simulink model "NonlinearMPC_FL_CBFcontroller"  (R2026a)
settings: Solver=VariableStepAuto  StopTime=120
PreLoadFcn:
  | % Define variants
  | VSS_PATH_CTRL_PURE_PURSUIT=Simulink.Variant('VSS_PATH_CTRL_MODE==1');
  | VSS_PATH_CTRL_REAR_WHEEL=Simulink.Variant('VSS_PATH_CTRL_MODE==2');
  | % Select default variant
  | VSS_PATH_CTRL_MODE =1;
  | 
  | 
  | % Longitudinal PID
  | LongitudinalPID.Kp = 20;
  | LongitudinalPID.Ki = 0;
  | LongitudinalPID.Kd = 0;
  | LongitudinalPID.N = 100;
  | LongitudinalPID.MaxAccel = 80;
  | LongitudinalPID.SampleTime = 0.01;
  | 
  | % Steering PID
  | SteeringPID.Kp = 60;
  | SteeringPID.Ki = 0;
  | SteeringPID.Kd = 5;
  | SteeringPID.N = 10;
  | SteeringPID.MaxSpeed =  10;
  | SteeringPID.MinSpeed = -10;
  | SteeringPID.SampleTime = 0.01;
  | 
  | 
  | 
  | setSMVehicleVisuParameters;
  | 
  | % Load planner commands
  | load('PlannerCmdTests.mat');
  | % Assign one for testing:
  | plannerCmd = plannerCmdFwd;
  | % plannerCmd  = plannerCmdFwdBwd;
  | 
  | % Bus structure definition
  | load('PlannerBusStruct.mat');
  | 
  | % Rear Wheel Controller Parameters
  | RW.k_e = 0.2;    % 0.1
  | RW.k_theta = 1;   % 0.75
  | RW.SampleTime =  0.1;
  | RW.GoalRadius = 0.3;
  | 
  | % Pure pursuit parameters
  | PP.DesiredLinearVel = 5;
  | PP.MaxAngularVel  = 10;
  | PP.LookaheadDist  = 1;
  | PP.Wheelbase = 4;
  | PP.GoalRadius = 0.1;
  | PP.SampleTime = 0.1;
  | PP.LongitudinalPID.Kp = 20;
  | PP.LongitudinalPID.Ki = 0;
  | PP.LongitudinalPID.Kd = 0;
  | PP.LongitudinalPID.N = 100;
  | PP.LongitudinalPID.MaxLongAccel =  80;
  | PP.LongitudinalPID.MinLongAccel = -80;
  | 
  | % Spline ref
  | splineRef = [ 0 0 0;[plannerCmd.PathMatrix(1:plannerCmd.PathLengths(1),1:2,1),0*ones(length(plannerCmd.PathMatrix(1:plannerCmd.PathLengths(1),1,1)),1)]];
values from neighbouring files (symbols this model uses):
  m = max(2, ceil(Lseg/ds))    [Trajectory.m]    (also in plot_nmpc_result.m = NaN)
  s = [0; cumsum(hypot(diff(xs),diff(ys)))]    [Trajectory.m]    (also in plot_parking_mpc.m = evalin('base',name); plot_result.m = out.(names{k}))
  trajMatrix = [tvec, xd, yd, thd, vd, wd]    [Trajectory.m]    (also in plot_parking_mpc.m = evalin('base','trajMatrix'); plot_result.m = evalin('base','trajMatrix'))
undefined symbols (not defined in the file or in its folder): DiscIntNeverNeededParam, smvv, X, Y, Z
libraries: sm_lib x527, sm_vehicle_slalom_lib x48, fl_lib x40, fl_ps_legacy_lib x28, nesl_utility x13
(part 15 of 15)

== system NonlinearMPC_FL_CBFcontroller/Robot Bicycle Model/Visualizer/SM_Car_Visu/Vehicle7/Steering_Wheel/Logo/LStick3 ==
  Stick : sm_lib/Body Elements/Brick Solid  BrickDimensions=[smvv.steeringwheel.letterStick 0.001 0.001]  BrickDimensionsUnits=m  ExportEntireGeometry=off  InertiaType=PointMass  BasedOnType=Density  Density=1000  DensityUnits=kg/m^3  Mass=0.001  MassUnits=kg  CenterOfMass=[0 0 0]  CenterOfMassUnits=m  MomentsOfInertia=[1 1 1]  MomentsOfInertiaUnits=kg*m^2  ProductsOfInertia=[1 1 1]  ProductsOfInertiaUnits=kg*m^2  GraphicType=FromGeometry  MarkerShape=Sphere  MarkerSize=10  GraphicVisPropType=SimpleVisualProperties  GraphicDiffuseColor=smvv.steeringwheel.letterColor  GraphicOpacity=1.0  GraphicSpecularColor=[0.5 0.5 0.5 1.0]  GraphicAmbientColor=[0.15 0.15 0.15 1.0]  GraphicEmissiveColor=[0.0 0.0 0.0 1.0]  GraphicShininess=75  DoExposeReferenceFrame=on  SerializedFrames=<Frames/>
  X offset 1 : sm_lib/Frames and Transforms/Rigid Transform  RotationMethod=None  FollAlignAxisA=+X  BaseAlignAxisA=+Y  FollAlignAxisB=+Y  BaseAlignAxisB=+Z  RotationStandardAxis=+X  RotationAngle=0  RotationAngleUnits=deg  RotationArbitraryAxis=[0 0 1]  RotationSequenceAxes=FollowerAxes  RotationSequence=XYX  RotationSequenceAngles=[0 0 0]  RotationSequenceAnglesUnits=deg  RotationMatrix=[1 0 0; 0 1 0; 0 0 1]  Quaternion=[1 0 0 0]  TranslationMethod=StandardAxis  TranslationCartesianOffset=[0 0 0]  TranslationCartesianOffsetUnits=m  TranslationStandardAxis=-X  TranslationStandardOffset=0.5*smvv.steeringwheel.letterStick  TranslationStandardOffsetUnits=m  TranslationROffset=0  TranslationROffsetUnits=m  TranslationThetaOffset=0  TranslationThetaOffsetUnits=deg  TranslationZOffset=0  TranslationZOffsetUnits=m
  x offset 2 : sm_lib/Frames and Transforms/Rigid Transform  RotationMethod=None  FollAlignAxisA=+X  BaseAlignAxisA=+Y  FollAlignAxisB=+Y  BaseAlignAxisB=+Z  RotationStandardAxis=+X  RotationAngle=0  RotationAngleUnits=deg  RotationArbitraryAxis=[0 0 1]  RotationSequenceAxes=FollowerAxes  RotationSequence=XYX  RotationSequenceAngles=[0 0 0]  RotationSequenceAnglesUnits=deg  RotationMatrix=[1 0 0; 0 1 0; 0 0 1]  Quaternion=[1 0 0 0]  TranslationMethod=StandardAxis  TranslationCartesianOffset=[0 0 0]  TranslationCartesianOffsetUnits=m  TranslationStandardAxis=+X  TranslationStandardOffset=0.5*smvv.steeringwheel.letterStick  TranslationStandardOffsetUnits=m  TranslationROffset=0  TranslationROffsetUnits=m  TranslationThetaOffset=0  TranslationThetaOffsetUnits=deg  TranslationZOffset=0  TranslationZOffsetUnits=m
  Conn1 : PMIOPort  Side=Left
  Conn2 : PMIOPort  Port=2  Side=Right
  connections:
  X offset 1/RConn1 -- Conn1/RConn1
  x offset 2/RConn1 -- Conn2/RConn1
  x offset 2/LConn1 -- Stick/RConn1 -- X offset 1/LConn1

== system NonlinearMPC_FL_CBFcontroller/Robot Bicycle Model/Visualizer/SM_Car_Visu/Vehicle7/Steering_Wheel/Logo/LStick4 ==
  Stick : sm_lib/Body Elements/Brick Solid  BrickDimensions=[smvv.steeringwheel.letterStick 0.001 0.001]  BrickDimensionsUnits=m  ExportEntireGeometry=off  InertiaType=PointMass  BasedOnType=Density  Density=1000  DensityUnits=kg/m^3  Mass=0.001  MassUnits=kg  CenterOfMass=[0 0 0]  CenterOfMassUnits=m  MomentsOfInertia=[1 1 1]  MomentsOfInertiaUnits=kg*m^2  ProductsOfInertia=[1 1 1]  ProductsOfInertiaUnits=kg*m^2  GraphicType=FromGeometry  MarkerShape=Sphere  MarkerSize=10  GraphicVisPropType=SimpleVisualProperties  GraphicDiffuseColor=smvv.steeringwheel.letterColor  GraphicOpacity=1.0  GraphicSpecularColor=[0.5 0.5 0.5 1.0]  GraphicAmbientColor=[0.15 0.15 0.15 1.0]  GraphicEmissiveColor=[0.0 0.0 0.0 1.0]  GraphicShininess=75  DoExposeReferenceFrame=on  SerializedFrames=<Frames/>
  X offset 1 : sm_lib/Frames and Transforms/Rigid Transform  RotationMethod=None  FollAlignAxisA=+X  BaseAlignAxisA=+Y  FollAlignAxisB=+Y  BaseAlignAxisB=+Z  RotationStandardAxis=+X  RotationAngle=0  RotationAngleUnits=deg  RotationArbitraryAxis=[0 0 1]  RotationSequenceAxes=FollowerAxes  RotationSequence=XYX  RotationSequenceAngles=[0 0 0]  RotationSequenceAnglesUnits=deg  RotationMatrix=[1 0 0; 0 1 0; 0 0 1]  Quaternion=[1 0 0 0]  TranslationMethod=StandardAxis  TranslationCartesianOffset=[0 0 0]  TranslationCartesianOffsetUnits=m  TranslationStandardAxis=-X  TranslationStandardOffset=0.5*smvv.steeringwheel.letterStick  TranslationStandardOffsetUnits=m  TranslationROffset=0  TranslationROffsetUnits=m  TranslationThetaOffset=0  TranslationThetaOffsetUnits=deg  TranslationZOffset=0  TranslationZOffsetUnits=m
  Conn1 : PMIOPort  Side=Left
  connections:
  Stick/RConn1 -- X offset 1/LConn1
  X offset 1/RConn1 -- Conn1/RConn1

== system NonlinearMPC_FL_CBFcontroller/Robot Bicycle Model/Visualizer/SM_Car_Visu/Vehicle7/Steering_Wheel/Logo/LStick5 ==
  Stick : sm_lib/Body Elements/Brick Solid  BrickDimensions=[smvv.steeringwheel.letterStick 0.001 0.001]  BrickDimensionsUnits=m  ExportEntireGeometry=off  InertiaType=PointMass  BasedOnType=Density  Density=1000  DensityUnits=kg/m^3  Mass=0.001  MassUnits=kg  CenterOfMass=[0 0 0]  CenterOfMassUnits=m  MomentsOfInertia=[1 1 1]  MomentsOfInertiaUnits=kg*m^2  ProductsOfInertia=[1 1 1]  ProductsOfInertiaUnits=kg*m^2  GraphicType=FromGeometry  MarkerShape=Sphere  MarkerSize=10  GraphicVisPropType=SimpleVisualProperties  GraphicDiffuseColor=smvv.steeringwheel.letterColor  GraphicOpacity=1.0  GraphicSpecularColor=[0.5 0.5 0.5 1.0]  GraphicAmbientColor=[0.15 0.15 0.15 1.0]  GraphicEmissiveColor=[0.0 0.0 0.0 1.0]  GraphicShininess=75  DoExposeReferenceFrame=on  SerializedFrames=<Frames/>
  X offset 1 : sm_lib/Frames and Transforms/Rigid Transform  RotationMethod=None  FollAlignAxisA=+X  BaseAlignAxisA=+Y  FollAlignAxisB=+Y  BaseAlignAxisB=+Z  RotationStandardAxis=+X  RotationAngle=0  RotationAngleUnits=deg  RotationArbitraryAxis=[0 0 1]  RotationSequenceAxes=FollowerAxes  RotationSequence=XYX  RotationSequenceAngles=[0 0 0]  RotationSequenceAnglesUnits=deg  RotationMatrix=[1 0 0; 0 1 0; 0 0 1]  Quaternion=[1 0 0 0]  TranslationMethod=StandardAxis  TranslationCartesianOffset=[0 0 0]  TranslationCartesianOffsetUnits=m  TranslationStandardAxis=-X  TranslationStandardOffset=0.5*smvv.steeringwheel.letterStick  TranslationStandardOffsetUnits=m  TranslationROffset=0  TranslationROffsetUnits=m  TranslationThetaOffset=0  TranslationThetaOffsetUnits=deg  TranslationZOffset=0  TranslationZOffsetUnits=m
  x offset 2 : sm_lib/Frames and Transforms/Rigid Transform  RotationMethod=None  FollAlignAxisA=+X  BaseAlignAxisA=+Y  FollAlignAxisB=+Y  BaseAlignAxisB=+Z  RotationStandardAxis=+X  RotationAngle=0  RotationAngleUnits=deg  RotationArbitraryAxis=[0 0 1]  RotationSequenceAxes=FollowerAxes  RotationSequence=XYX  RotationSequenceAngles=[0 0 0]  RotationSequenceAnglesUnits=deg  RotationMatrix=[1 0 0; 0 1 0; 0 0 1]  Quaternion=[1 0 0 0]  TranslationMethod=StandardAxis  TranslationCartesianOffset=[0 0 0]  TranslationCartesianOffsetUnits=m  TranslationStandardAxis=+X  TranslationStandardOffset=0.5*smvv.steeringwheel.letterStick  TranslationStandardOffsetUnits=m  TranslationROffset=0  TranslationROffsetUnits=m  TranslationThetaOffset=0  TranslationThetaOffsetUnits=deg  TranslationZOffset=0  TranslationZOffsetUnits=m
  Conn1 : PMIOPort  Side=Left
  Conn2 : PMIOPort  Port=2  Side=Right
  connections:
  X offset 1/RConn1 -- Conn1/RConn1
  x offset 2/RConn1 -- Conn2/RConn1
  x offset 2/LConn1 -- Stick/RConn1 -- X offset 1/LConn1

== system NonlinearMPC_FL_CBFcontroller/Robot Bicycle Model/Visualizer/SM_Car_Visu/Vehicle7/Steering_Wheel/Logo/LStick6 ==
  Stick : sm_lib/Body Elements/Brick Solid  BrickDimensions=[2*smvv.steeringwheel.letterStick 0.001 0.001]  BrickDimensionsUnits=m  ExportEntireGeometry=off  InertiaType=PointMass  BasedOnType=Density  Density=1000  DensityUnits=kg/m^3  Mass=0.001  MassUnits=kg  CenterOfMass=[0 0 0]  CenterOfMassUnits=m  MomentsOfInertia=[1 1 1]  MomentsOfInertiaUnits=kg*m^2  ProductsOfInertia=[1 1 1]  ProductsOfInertiaUnits=kg*m^2  GraphicType=FromGeometry  MarkerShape=Sphere  MarkerSize=10  GraphicVisPropType=SimpleVisualProperties  GraphicDiffuseColor=smvv.steeringwheel.letterColor  GraphicOpacity=1.0  GraphicSpecularColor=[0.5 0.5 0.5 1.0]  GraphicAmbientColor=[0.15 0.15 0.15 1.0]  GraphicEmissiveColor=[0.0 0.0 0.0 1.0]  GraphicShininess=75  DoExposeReferenceFrame=on  SerializedFrames=<Frames/>
  X offset 1 : sm_lib/Frames and Transforms/Rigid Transform  RotationMethod=None  FollAlignAxisA=+X  BaseAlignAxisA=+Y  FollAlignAxisB=+Y  BaseAlignAxisB=+Z  RotationStandardAxis=+X  RotationAngle=0  RotationAngleUnits=deg  RotationArbitraryAxis=[0 0 1]  RotationSequenceAxes=FollowerAxes  RotationSequence=XYX  RotationSequenceAngles=[0 0 0]  RotationSequenceAnglesUnits=deg  RotationMatrix=[1 0 0; 0 1 0; 0 0 1]  Quaternion=[1 0 0 0]  TranslationMethod=StandardAxis  TranslationCartesianOffset=[0 0 0]  TranslationCartesianOffsetUnits=m  TranslationStandardAxis=-X  TranslationStandardOffset=smvv.steeringwheel.letterStick  TranslationStandardOffsetUnits=m  TranslationROffset=0  TranslationROffsetUnits=m  TranslationThetaOffset=0  TranslationThetaOffsetUnits=deg  TranslationZOffset=0  TranslationZOffsetUnits=m
  x offset 2 : sm_lib/Frames and Transforms/Rigid Transform  RotationMethod=None  FollAlignAxisA=+X  BaseAlignAxisA=+Y  FollAlignAxisB=+Y  BaseAlignAxisB=+Z  RotationStandardAxis=+X  RotationAngle=0  RotationAngleUnits=deg  RotationArbitraryAxis=[0 0 1]  RotationSequenceAxes=FollowerAxes  RotationSequence=XYX  RotationSequenceAngles=[0 0 0]  RotationSequenceAnglesUnits=deg  RotationMatrix=[1 0 0; 0 1 0; 0 0 1]  Quaternion=[1 0 0 0]  TranslationMethod=StandardAxis  TranslationCartesianOffset=[0 0 0]  TranslationCartesianOffsetUnits=m  TranslationStandardAxis=+X  TranslationStandardOffset=smvv.steeringwheel.letterStick  TranslationStandardOffsetUnits=m  TranslationROffset=0  TranslationROffsetUnits=m  TranslationThetaOffset=0  TranslationThetaOffsetUnits=deg  TranslationZOffset=0  TranslationZOffsetUnits=m
  Conn1 : PMIOPort  Side=Left
  Conn2 : PMIOPort  Port=2  Side=Right
  connections:
  X offset 1/LConn1 -- Stick/RConn1 -- x offset 2/LConn1
  x offset 2/RConn1 -- Conn2/RConn1
  X offset 1/RConn1 -- Conn1/RConn1

== system NonlinearMPC_FL_CBFcontroller/Robot Bicycle Model/Visualizer/SM_Car_Visu/Vehicle7/Steering_Wheel/Logo/LStick7 ==
  Stick : sm_lib/Body Elements/Brick Solid  BrickDimensions=[smvv.steeringwheel.letterStick 0.001 0.001]  BrickDimensionsUnits=m  ExportEntireGeometry=off  InertiaType=PointMass  BasedOnType=Density  Density=1000  DensityUnits=kg/m^3  Mass=0.001  MassUnits=kg  CenterOfMass=[0 0 0]  CenterOfMassUnits=m  MomentsOfInertia=[1 1 1]  MomentsOfInertiaUnits=kg*m^2  ProductsOfInertia=[1 1 1]  ProductsOfInertiaUnits=kg*m^2  GraphicType=FromGeometry  MarkerShape=Sphere  MarkerSize=10  GraphicVisPropType=SimpleVisualProperties  GraphicDiffuseColor=smvv.steeringwheel.letterColor  GraphicOpacity=1.0  GraphicSpecularColor=[0.5 0.5 0.5 1.0]  GraphicAmbientColor=[0.15 0.15 0.15 1.0]  GraphicEmissiveColor=[0.0 0.0 0.0 1.0]  GraphicShininess=75  DoExposeReferenceFrame=on  SerializedFrames=<Frames/>
  X offset 1 : sm_lib/Frames and Transforms/Rigid Transform  RotationMethod=None  FollAlignAxisA=+X  BaseAlignAxisA=+Y  FollAlignAxisB=+Y  BaseAlignAxisB=+Z  RotationStandardAxis=+X  RotationAngle=0  RotationAngleUnits=deg  RotationArbitraryAxis=[0 0 1]  RotationSequenceAxes=FollowerAxes  RotationSequence=XYX  RotationSequenceAngles=[0 0 0]  RotationSequenceAnglesUnits=deg  RotationMatrix=[1 0 0; 0 1 0; 0 0 1]  Quaternion=[1 0 0 0]  TranslationMethod=StandardAxis  TranslationCartesianOffset=[0 0 0]  TranslationCartesianOffsetUnits=m  TranslationStandardAxis=-X  TranslationStandardOffset=0.5*smvv.steeringwheel.letterStick  TranslationStandardOffsetUnits=m  TranslationROffset=0  TranslationROffsetUnits=m  TranslationThetaOffset=0  TranslationThetaOffsetUnits=deg  TranslationZOffset=0  TranslationZOffsetUnits=m
  Conn1 : PMIOPort  Side=Left
  connections:
  X offset 1/RConn1 -- Conn1/RConn1
  Stick/RConn1 -- X offset 1/LConn1

== matlab function NonlinearMPC_FL_CBFcontroller/MATLAB Function1 ==
  data: pose input; v_out output; u1_cmd input; u2_cmd input; delta_out output; h_min_out output; qp_status output; h_red_out output; h_pink_out output; h_obs3_out output
function [v_out, delta_out, h_min_out, qp_status, ...
          h_red_out, h_pink_out, h_obs3_out] = ...
    fl_cbf_inner_filter_u1u2_reverse(pose, u1_cmd, u2_cmd)
% Fast feedback-linearization + CBF safety filter for the reverse-phase outer.
%
% Inputs u1_cmd and u2_cmd are the virtual velocity of the point
%   P = [x;y] + ell*[cos(theta);sin(theta)].
% This block converts them to q = [v; v*tan(delta)] and projects q into
% the CBF-safe and actuator-limited set.

coder.extrinsic('quadprog');
coder.extrinsic('optimoptions');

%% Parameters
% IMPORTANT: set this equal to the sample time of this MATLAB Function
% block. For a 100 Hz inner loop use 0.01; for 50 Hz use 0.02.
Ts = 0.01;

L        = 3.0;
ell      = L;
vMin     = -2.5;
vMax     =  3.0;
dMax     = 60*pi/180;
tanDMax  = tan(dMax);
aMax     = 3.0;
dRate    = 0.60;
gammaCBF = 0.30;

% Obstacle circles: [cx, cy, inflated radius].
obs = [53.5, 21.0, 3.64;   % red, rear  (unchanged)
    56.5, 21.0, 3.64;   % red, front (unchanged)
    37.5, 21.0, 3.64;   % pink, rear  ← FIX: was 38.5, should be 37.5
    40.5, 21.0, 3.64;   % pink, front (correct)
    26.6, 17.0, 3.24];  % obstacle 3  (unchanged)

nObs = 5;

%% Persistent actuator state and gear hysteresis
persistent prevV prevDelta gear

if isempty(prevV) || isempty(prevDelta) || isempty(gear)
    prevV     = 0.0;
    prevDelta = 0.0;
    gear      = 1.0;
end

pose = double(pose(:));
pose = pose(1:3);
pose(3) = atan2(sin(pose(3)),cos(pose(3)));

uRef = [double(u1_cmd);double(u2_cmd)];

th = pose(3);
eTheta = [cos(th);sin(th)];
ePerp  = [-sin(th);cos(th)];

% P_dot = eTheta*v + (ell/L)*ePerp*(v*tan(delta)).
% Therefore:
%   v          = eTheta.'*uRef
%   v*tan(del) = (L/ell)*ePerp.'*uRef
vNom  = eTheta.'*uRef;
q2Nom = (L/ell)*(ePerp.'*uRef);
vNom  = max(vMin,min(vMax,vNom));

% Gear hysteresis prevents rapid switching between forward and reverse
% steering cones when the planned longitudinal velocity crosses zero.
if gear >= 0.0
    if vNom < -0.15
        gear = -1.0;
    end
else
    if vNom > 0.15
        gear = 1.0;
    end
end

if abs(vNom) <= 0.15 && abs(prevV) > 0.20
    gear = sign(prevV);
end

%% Current barrier diagnostics
hRedOut = minimumBarrierAgainstSet(pose,obs(1:2,:),L);
hPinkOut = minimumBarrierAgainstSet(pose,obs(3:4,:),L);
hObs3Out = minimumBarrierAgainstSet(pose,obs(5:5,:),L);

h_red_out  = hRedOut;
h_pink_out = hPinkOut;
h_obs3_out = hObs3Out;
h_min_out  = min(hRedOut,min(hPinkOut,hObs3Out));

%% Nominal auxiliary input obtained from feedback linearization
qNom = [vNom;q2Nom];

% Penalize changes in velocity more than changes in the auxiliary steering
% variable. The exact steering wheel is recovered after the QP.
wV = 8.0;
wQ = 2.0;

H = diag([2.0*wV,2.0*wQ]);
f = [-2.0*wV*qNom(1);
     -2.0*wQ*qNom(2)];

% Suppress repeated solver messages in the Simulation Diagnostics window.
qpOptions = optimoptions('quadprog', ...
    'Algorithm','interior-point-convex','Display','off');

%% Bounds and actuator-rate limits
dvMax = aMax*Ts;
ddMax = dRate*Ts;

q2Prev = prevV*tan(prevDelta);

% This box is a conservative linear approximation of steering-rate
% limiting in q-space.
dq2Max = abs(prevV)*ddMax + dvMax*tanDMax + 0.02;

lb = [max(vMin,prevV-dvMax);
      max(-vMax*tanDMax,q2Prev-dq2Max)];

ub = [min(vMax,prevV+dvMax);
      min( vMax*tanDMax,q2Prev+dq2Max)];

%% Try the selected gear cone first, then the opposite cone if necessary
qSol       = [0.0;0.0];
exitStatus = -100.0;
solved     = false;
usedGear   = gear;

for attempt = 1:2
    if attempt == 1
        gearTry = gear;
    else
        gearTry = -gear;
    end

    Aineq = zeros(2*nObs+2,2);
    bineq = zeros(2*nObs+2,1);
    row = 0;

    % Exact sufficient linear DCBF constraints for both ego circles.
    for j = 1:nObs
        cx = obs(j,1);
        cy = obs(j,2);
        rr = obs(j,3);

        [hRear,aRear] = rearCbfRow(pose,cx,cy,rr,Ts);
        row = row+1;
        Aineq(row,:) = aRear.';
        bineq(row)   = gammaCBF*hRear;

        [hFront,aFront] = frontCbfRow(pose,cx,cy,rr,Ts,L);
        row = row+1;
        Aineq(row,:) = aFront.';
        bineq(row)   = gammaCBF*hFront;
    end

    % Steering cone. Because q2=v*tan(delta), the feasible steering cone
    % depends on the direction of motion.
    if gearTry >= 0.0
        % Forward: |q2| <= tan(dMax)*q1. This also enforces q1 >= 0.
        row = row+1;
        Aineq(row,:) = [-tanDMax,  1.0];
        bineq(row)   = 0.0;

        row = row+1;
        Aineq(row,:) = [-tanDMax, -1.0];
        bineq(row)   = 0.0;
    else
        % Reverse: tan(dMax)*q1 <= q2 <= -tan(dMax)*q1.
        % This also enforces q1 <= 0.
        row = row+1;
        Aineq(row,:) = [tanDMax,  1.0];
        bineq(row)   = 0.0;

        row = row+1;
        Aineq(row,:) = [tanDMax, -1.0];
        bineq(row)   = 0.0;
    end

    % quadprog returns an empty q when it declares the QP infeasible.
    % Keep the raw output variable-size and copy only after checking its
    % length, preventing a 2x1 versus 0x0 runtime mismatch.
    qTryRaw = zeros(0,1);
    coder.varsize('qTryRaw',[2 1],[true false]);
    exitTry = 0.0;

    [qTryRaw,~,exitTry] = quadprog( ...
        H,f,Aineq,bineq,[],[],lb,ub,[],qpOptions);

    qTry = zeros(2,1);
    qTryOK = false;

    if exitTry > 0 && size(qTryRaw,1) == 2
        qTry(:) = qTryRaw(1:2);
        qTryOK = true;

        if ~isfinite(qTry(1)) || ~isfinite(qTry(2))
            qTryOK = false;
        end
    end

    if qTryOK
        qSol       = qTry;
        exitStatus = exitTry;
        solved     = true;
        usedGear   = gearTry;
        break;
    end
end

%% Convert auxiliary input to actuator commands
if solved
    vOut = qSol(1);

    if abs(vOut) < 1e-4
        vOut     = 0.0;
        deltaOut = prevDelta;
    else
        deltaOut = atan(qSol(2)/vOut);
    end

    vOut     = max(vMin,min(vMax,vOut));
    deltaOut = max(-dMax,min(dMax,deltaOut));

    % Keep the persistent cone consistent with the successful QP cone.
    gear = usedGear;
else
    % If both cones are infeasible, stop. If the current state is safe,
    % zero velocity keeps the one-step state inside the safe set.
    vOut       = 0.0;
    deltaOut   = prevDelta;
    exitStatus = -10.0;
end

v_out     = vOut;
delta_out = deltaOut;
qp_status = exitStatus;

prevV     = v_out;
prevDelta = delta_out;

end

%% -----------------------------------------------------------------------
function hMin = minimumBarrierAgainstSet(x,obsSet,L)

nLocal = size(obsSet,1);
hMin = 1.0e12;

for j = 1:nLocal
    cx = obsSet(j,1);
    cy = obsSet(j,2);
    rr = obsSet(j,3);

    hRear = rearBarrier(x,cx,cy,rr);
    hFront = frontBarrier(x,cx,cy,rr,L);
    hBoth = min(hRear,hFront);

    if hBoth < hMin
        hMin = hBoth;
    end
end

end

%% -----------------------------------------------------------------------
function h = rearBarrier(x,cx,cy,r)

dx = x(1)-cx;
dy = x(2)-cy;
h  = dx*dx+dy*dy-r*r;

end

%% -----------------------------------------------------------------------
function h = frontBarrier(x,cx,cy,r,L)

th = x(3);
px = x(1)+L*cos(th);
py = x(2)+L*sin(th);

dx = px-cx;
dy = py-cy;
h  = dx*dx+dy*dy-r*r;

end

%% -----------------------------------------------------------------------
function [h,a] = rearCbfRow(x,cx,cy,r,Ts)
% Rear ego center moves as p_next = p + Ts*e*q1.
% h_next = h + 2*d'*G*q + ||G*q||^2, so
% 2*d'*G*q >= -gamma*h is sufficient for h_next >= (1-gamma)*h.

th = x(3);
e = [cos(th);sin(th)];

d = [x(1)-cx;
     x(2)-cy];

h = d.'*d-r*r;

G = [Ts*e, zeros(2,1)];

% We need 2*d'*G*q >= -gamma*h, i.e. -2*d'*G*q <= gamma*h.
a = -2.0*(d.'*G).';

end

%% -----------------------------------------------------------------------
function [h,a] = frontCbfRow(x,cx,cy,r,Ts,L)
% Front ego center moves as
% p_next = p + Ts*e*q1 + Ts*e_perp*q2,
% where q2 = v*tan(delta).

th = x(3);
e     = [cos(th);sin(th)];
ePerp = [-sin(th);cos(th)];

px = x(1)+L*cos(th);
py = x(2)+L*sin(th);

d = [px-cx;
     py-cy];

h = d.'*d-r*r;

G = Ts*[e,ePerp];

a = -2.0*(d.'*G).';

end

== matlab function NonlinearMPC_FL_CBFcontroller/MATLAB Function ==
  data: pose input; trajectory input; u1_cmd output; t input; u2_cmd output; P_pred_out output; qp_status output; scp_passes_out output; mode_out output; qp_inner input; solve_ms output
function [u1_cmd, u2_cmd, P_pred_out, qp_status, scp_passes_out, mode_out, solve_ms] = ...
    fcn(pose, trajectory, t, qp_inner)

coder.extrinsic('mpc_outer_fmincon_nmpc');

% Predeclare outputs with the correct types/sizes
u1_cmd         = 0.0;
u2_cmd         = 0.0;
P_pred_out     = zeros(2,6);   % 2 x (Np+1)  -- Np = 5 in the .m file
qp_status      = 0.0;
scp_passes_out = 0.0;
mode_out       = 1.0;
solve_ms       = 0.0;

[u1_cmd, u2_cmd, P_pred_out, qp_status, scp_passes_out, mode_out, solve_ms] = ...
    mpc_outer_fmincon_nmpc(pose, trajectory, t, qp_inner);
end

== matlab function NonlinearMPC_FL_CBFcontroller/Robot Bicycle Model/wrapToPi ==
  data: qIn input; qOut output
function qOut = wrapToPi(qIn)
%#codegen

qOut = angdiff(0*qIn, qIn);
